simulink model "ATOM_simple_planning_simulator"  (R2026a)
settings: Solver=ode4  StopTime=50  FixedStep=0.01
StopFcn:
  | if exist('costmap_active','var') && ...
  |    exist('vehicle','var') && ...
  |    exist('parking_path','var') && ...
  |    ~isempty(parking_path)
  | 
  |     plotPlan(costmap_active, vehicle, parking_path);
  | else
  |     warning('No valid parking path is available for plotting.');
  | end
model workspace (MAT data in the model file):
  vehicle : object (value not decoded)
symbols that are objects in the model workspace (value not decoded): vehicle
undefined symbols (not defined in the file or in its folder): delta_f_LUT, gain4WS_LUT, k_ref_LUT, kappa_gain_BP, Ki, Kp, lateral, longitudinal, planning_validator, rr_gain_BP, rr_LUT, stanley, velocity_smoother
libraries: slpidlib x1, simulink x1
(part 2 of 7)

== system ATOM_simple_planning_simulator/Parking Scenario/Costmap generation: perpendicular lot ==
  From Workspace1 : FromWorkspace  VariableName=veh
  Perpendicular Parking : MATLAB Function  TreatAsAtomicUnit=on
  costmap : Outport
  start_pose : Outport  Port=2
  goal_pose : Outport  Port=3
  wires:
  Perpendicular Parking/1(costmap) -> costmap/1
  From Workspace1/1 -> Perpendicular Parking/1(veh)
  Perpendicular Parking/2(start_pose) -> start_pose/1
  Perpendicular Parking/3(goal_pose) -> goal_pose/1

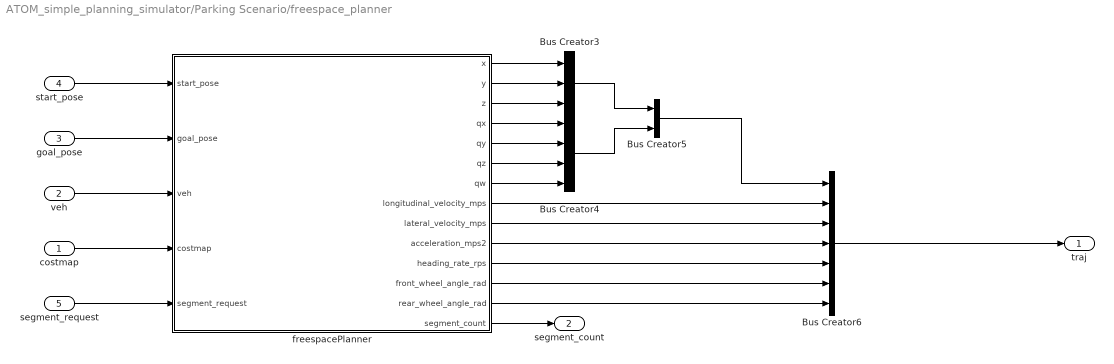
== system ATOM_simple_planning_simulator/Parking Scenario/freespace_planner ==
  costmap : Inport
  veh : Inport  Port=2
  goal_pose : Inport  Port=3
  start_pose : Inport  Port=4
  segment_request : Inport  Port=5
  Bus Creator3 : BusCreator  Inputs=3  OutDataTypeStr=Bus: PointBusN
  Bus Creator4 : BusCreator  Inputs=4  OutDataTypeStr=Bus: QuaternionBusN
  Bus Creator5 : BusCreator  Inputs=2  OutDataTypeStr=Bus: PoseBusN
      settings: InheritFromInputs=off
  Bus Creator6 : BusCreator  Inputs=7  OutDataTypeStr=Bus: TrajectoryDataBus
      settings: InheritFromInputs=off
  freespacePlanner : MATLAB Function  TreatAsAtomicUnit=on
  traj : Outport
  segment_count : Outport  Port=2
  wires:
  Bus Creator6/1 -> traj/1
  Bus Creator3/1 -> Bus Creator5/1
  freespacePlanner/13(rear_wheel_angle_rad) -> Bus Creator6/7
  Bus Creator5/1 -> Bus Creator6/1
  freespacePlanner/8(longitudinal_velocity_mps) -> Bus Creator6/2
  freespacePlanner/3(z) -> Bus Creator3/3
  freespacePlanner/4(qx) -> Bus Creator4/1
  freespacePlanner/9(lateral_velocity_mps) -> Bus Creator6/3
  freespacePlanner/10(acceleration_mps2) -> Bus Creator6/4
  freespacePlanner/5(qy) -> Bus Creator4/2
  freespacePlanner/1(x) -> Bus Creator3/1
  freespacePlanner/2(y) -> Bus Creator3/2
  freespacePlanner/7(qw) -> Bus Creator4/4
  freespacePlanner/6(qz) -> Bus Creator4/3
  freespacePlanner/12(front_wheel_angle_rad) -> Bus Creator6/6
  Bus Creator4/1 -> Bus Creator5/2
  freespacePlanner/11(heading_rate_rps) -> Bus Creator6/5
  costmap/1 -> freespacePlanner/4(costmap)
  start_pose/1 -> freespacePlanner/1(start_pose)
  goal_pose/1 -> freespacePlanner/2(goal_pose)
  veh/1 -> freespacePlanner/3(veh)
  segment_request/1 -> freespacePlanner/5(segment_request)
  freespacePlanner/14(segment_count) -> segment_count/1

== system ATOM_simple_planning_simulator/Plot vehicle/SetStanleyTrajectory ==
  ref_traj : Inport
  ego_pose : Inport  Port=2
  Constant1 : Constant  Value=stanley.traj_resample_dist
  Resample Trajectory : MATLAB Function  TreatAsAtomicUnit=on
  calcLongOffsetToSegment : MATLAB Function  TreatAsAtomicUnit=on
  default : Constant  Value=3
  default1 : Constant  Value=pi/2
  findFirstNearestSegmentIndexWithSoftConstraints : MATLAB Function  TreatAsAtomicUnit=on
  trajectory_out : Outport
  wires:
  ref_traj/1 -> Resample Trajectory/1(trajectory_in), calcLongOffsetToSegment/3(trajectory), findFirstNearestSegmentIndexWithSoftConstraints/1(trajectory)
  Constant1/1 -> Resample Trajectory/2(resample_interval_dist)
  calcLongOffsetToSegment/1(ego_offset_to_segment) -> Resample Trajectory/4(ego_offset_to_segment)
  ego_pose/1 -> findFirstNearestSegmentIndexWithSoftConstraints/4(pose), calcLongOffsetToSegment/2(ego_pose)
  findFirstNearestSegmentIndexWithSoftConstraints/1(nearest_seg_idx) -> calcLongOffsetToSegment/1(seg_idx), Resample Trajectory/3(nearest_seg_idx)
  default/1 -> findFirstNearestSegmentIndexWithSoftConstraints/2(dist_threshold)
  default1/1 -> findFirstNearestSegmentIndexWithSoftConstraints/3(yaw_threshold)
  Resample Trajectory/1(trajectory_out) -> trajectory_out/1

== system ATOM_simple_planning_simulator/Plot vehicle1/SetStanleyTrajectory ==
  ref_traj : Inport
  ego_pose : Inport  Port=2
  Constant1 : Constant  Value=stanley.traj_resample_dist
  Resample Trajectory : MATLAB Function  TreatAsAtomicUnit=on
  calcLongOffsetToSegment : MATLAB Function  TreatAsAtomicUnit=on
  default : Constant  Value=3
  default1 : Constant  Value=pi/2
  findFirstNearestSegmentIndexWithSoftConstraints : MATLAB Function  TreatAsAtomicUnit=on
  trajectory_out : Outport
  wires:
  ref_traj/1 -> Resample Trajectory/1(trajectory_in), calcLongOffsetToSegment/3(trajectory), findFirstNearestSegmentIndexWithSoftConstraints/1(trajectory)
  Constant1/1 -> Resample Trajectory/2(resample_interval_dist)
  calcLongOffsetToSegment/1(ego_offset_to_segment) -> Resample Trajectory/4(ego_offset_to_segment)
  ego_pose/1 -> findFirstNearestSegmentIndexWithSoftConstraints/4(pose), calcLongOffsetToSegment/2(ego_pose)
  findFirstNearestSegmentIndexWithSoftConstraints/1(nearest_seg_idx) -> calcLongOffsetToSegment/1(seg_idx), Resample Trajectory/3(nearest_seg_idx)
  default/1 -> findFirstNearestSegmentIndexWithSoftConstraints/2(dist_threshold)
  default1/1 -> findFirstNearestSegmentIndexWithSoftConstraints/3(yaw_threshold)
  Resample Trajectory/1(trajectory_out) -> trajectory_out/1

== system ATOM_simple_planning_simulator/Vehicle Model/Vehicle Dynamics ==
  command : Inport
  rear_steer_command : Inport  Port=2
  From Workspace : FromWorkspace  VariableName=veh
  MATLAB Function : MATLAB Function  TreatAsAtomicUnit=on
  state integrator : Subsystem
  IntState : Outport
  wires:
  command/1 -> MATLAB Function/2(command)
  MATLAB Function/1(d_state) -> state integrator/1(d_state)  "d_state"
  state integrator/1(state) -> MATLAB Function/1(state), IntState/1
  From Workspace/1 -> MATLAB Function/3(veh)
  rear_steer_command/1 -> MATLAB Function/4(rear_steering_command)

== system ATOM_simple_planning_simulator/Vehicle Model/Vehicle internal state ==
  IntState : Inport
  Bus Selector : BusSelector  OutputSignals=x,y,yaw,vx,steer_front,steer_rear,acc
  Scope{,1..6} (7 alike) : Scope
      Scope settings: ActiveDisplayYMinimum=-1  ActiveDisplayYMaximum=1
      Scope1 settings: ActiveDisplayYMinimum=-1  ActiveDisplayYMaximum=1
      Scope2 settings: ActiveDisplayYMinimum=-1  ActiveDisplayYMaximum=1  DataLoggingVariableName=ScopeData2
      Scope3 settings: ActiveDisplayYMinimum=-1  ActiveDisplayYMaximum=1  DataLoggingVariableName=ScopeData3
      Scope4 settings: ActiveDisplayYMinimum=-1  ActiveDisplayYMaximum=1  DataLoggingVariableName=ScopeData4
      Scope5 settings: ActiveDisplayYMinimum=-1  ActiveDisplayYMaximum=1  DataLoggingVariableName=ScopeData5
      Scope6 settings: ActiveDisplayYMinimum=-1  ActiveDisplayYMaximum=1  DataLoggingVariableName=ScopeData6
  steer_front : Outport
  steer_rear : Outport  Port=2
  wires:
  Bus Selector/2 -> Scope1/1  "<y>"
  Bus Selector/4 -> Scope3/1  "<vx>"
  Bus Selector/1 -> Scope/1  "<x>"
  Bus Selector/3 -> Scope2/1  "<yaw>"
  Bus Selector/7 -> Scope6/1  "<acc>"
  Bus Selector/5 -> steer_front/1, Scope4/1  "<steer_front>"
  Bus Selector/6 -> steer_rear/1, Scope5/1  "<steer_rear>"
  IntState/1 -> Bus Selector/1

== system ATOM_simple_planning_simulator/Vehicle_Model/Vehicle Dynamics ==
  command : Inport
  rear_steer_command : Inport  Port=2
  From Workspace : FromWorkspace  VariableName=veh
  MATLAB Function : MATLAB Function  TreatAsAtomicUnit=on
  state integrator : Subsystem
  IntState : Outport
  wires:
  command/1 -> MATLAB Function/2(command)
  MATLAB Function/1(d_state) -> state integrator/1(d_state)  "d_state"
  state integrator/1(state) -> MATLAB Function/1(state), IntState/1
  From Workspace/1 -> MATLAB Function/3(veh)
  rear_steer_command/1 -> MATLAB Function/4(rear_steering_command)

== system ATOM_simple_planning_simulator/Vehicle_Model/Vehicle internal state ==
  IntState : Inport
  Bus Selector : BusSelector  OutputSignals=x,y,yaw,vx,steer_front,steer_rear,acc
  Scope{,1..6} (7 alike) : Scope
      Scope settings: ActiveDisplayYMinimum=-1  ActiveDisplayYMaximum=1
      Scope1 settings: ActiveDisplayYMinimum=-1  ActiveDisplayYMaximum=1
      Scope2 settings: ActiveDisplayYMinimum=-1  ActiveDisplayYMaximum=1  DataLoggingVariableName=ScopeData2
      Scope3 settings: ActiveDisplayYMinimum=-1  ActiveDisplayYMaximum=1  DataLoggingVariableName=ScopeData3
      Scope4 settings: ActiveDisplayYMinimum=-1  ActiveDisplayYMaximum=1  DataLoggingVariableName=ScopeData4
      Scope5 settings: ActiveDisplayYMinimum=-1  ActiveDisplayYMaximum=1  DataLoggingVariableName=ScopeData5
      Scope6 settings: ActiveDisplayYMinimum=-1  ActiveDisplayYMaximum=1  DataLoggingVariableName=ScopeData6
  steer_front : Outport
  steer_rear : Outport  Port=2
  wires:
  Bus Selector/2 -> Scope1/1  "<y>"
  Bus Selector/4 -> Scope3/1  "<vx>"
  Bus Selector/1 -> Scope/1  "<x>"
  Bus Selector/3 -> Scope2/1  "<yaw>"
  Bus Selector/7 -> Scope6/1  "<acc>"
  Bus Selector/5 -> steer_front/1, Scope4/1  "<steer_front>"
  Bus Selector/6 -> steer_rear/1, Scope5/1  "<steer_rear>"
  IntState/1 -> Bus Selector/1

== system ATOM_simple_planning_simulator/trajectory_checker plugin - planning_validator_node/check_valid_steering ==
  trajectory : Inport
  veh : Inport  Port=2
  CheckValidSteering : MATLAB Function  TreatAsAtomicUnit=on
  Constant : Constant  Value=planning_validator.steering.threshold
  calcMaxSteeringAngles : Subsystem
  is_valid_steering : Outport
  wires:
  calcMaxSteeringAngles/1(max_steering) -> CheckValidSteering/1(max_steering)
  calcMaxSteeringAngles/2(i) -> ?
  Constant/1 -> CheckValidSteering/2(steering_threshold)
  CheckValidSteering/1(is_valid_steering) -> is_valid_steering/1
  trajectory/1 -> calcMaxSteeringAngles/1(trajectory)
  veh/1 -> calcMaxSteeringAngles/2(veh)

== system ATOM_simple_planning_simulator/trajectory_checker plugin - planning_validator_node/check_valid_steering_rate ==
  trajectory : Inport
  veh : Inport  Port=2
  CheckValidSteeringRate : MATLAB Function  TreatAsAtomicUnit=on
  Constant : Constant  Value=planning_validator.steering_rate.threshold
  calcMaxSteeringRates : Subsystem
  is_valid_steering_rate : Outport
  wires:
  calcMaxSteeringRates/1(max_steering_rate) -> CheckValidSteeringRate/1(max_steering_rate)
  calcMaxSteeringRates/2(i) -> ?
  Constant/1 -> CheckValidSteeringRate/2(steering_rate_threshold)
  CheckValidSteeringRate/1(is_valid_steering_rate) -> is_valid_steering_rate/1
  trajectory/1 -> calcMaxSteeringRates/1(trajectory)
  veh/1 -> calcMaxSteeringRates/2(veh)

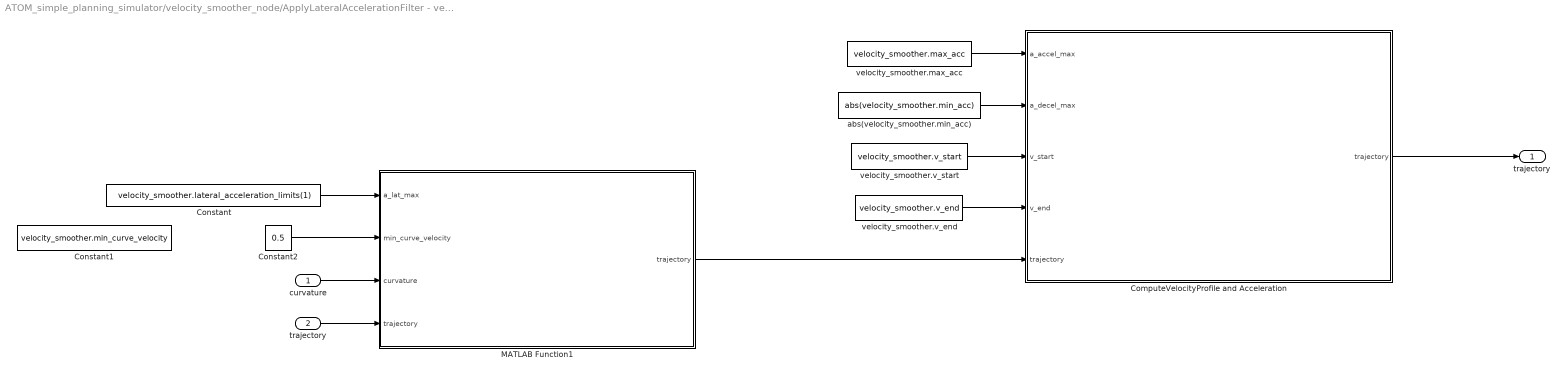
== system ATOM_simple_planning_simulator/velocity_smoother_node/ApplyLateralAccelerationFilter - velocity_smoother node ==
  curvature : Inport
  "trajectory " : Inport  Port=2
  ComputeVelocityProfile and Acceleration : MATLAB Function  TreatAsAtomicUnit=on
  Constant : Constant  Value=velocity_smoother.lateral_acceleration_limits(1)
  Constant1 : Constant  Value=velocity_smoother.min_curve_velocity
  Constant2 : Constant  Value=0.5
  MATLAB Function1 : MATLAB Function  TreatAsAtomicUnit=on
  abs(velocity_smoother.min_acc) : Constant  Value=abs(velocity_smoother.min_acc)
  velocity_smoother.max_acc : Constant  Value=velocity_smoother.max_acc
  velocity_smoother.v_end : Constant  Value=velocity_smoother.v_end
  velocity_smoother.v_start : Constant  Value=velocity_smoother.v_start
  trajectory : Outport
  wires:
  velocity_smoother.v_end/1 -> ComputeVelocityProfile and Acceleration/4(v_end)
  ComputeVelocityProfile and Acceleration/1(trajectory) -> trajectory/1
  curvature/1 -> MATLAB Function1/3(curvature)
  velocity_smoother.v_start/1 -> ComputeVelocityProfile and Acceleration/3(v_start)
  velocity_smoother.max_acc/1 -> ComputeVelocityProfile and Acceleration/1(a_accel_max)
  abs(velocity_smoother.min_acc)/1 -> ComputeVelocityProfile and Acceleration/2(a_decel_max)
  MATLAB Function1/1(trajectory) -> ComputeVelocityProfile and Acceleration/5("trajectory ")
  Constant2/1 -> MATLAB Function1/2(min_curve_velocity)
  Constant/1 -> MATLAB Function1/1(a_lat_max)
  "trajectory "/1 -> MATLAB Function1/4("trajectory ")

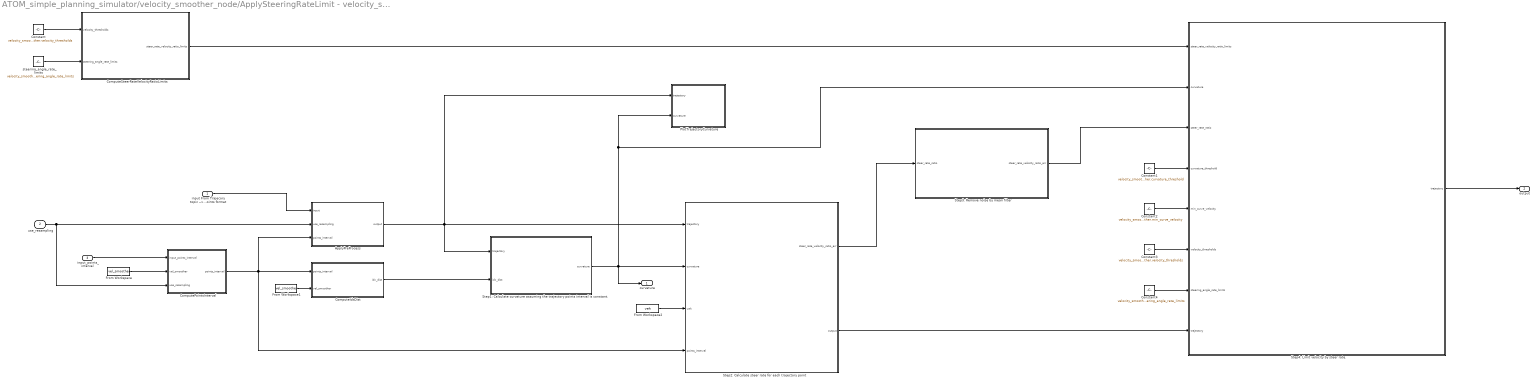
== system ATOM_simple_planning_simulator/velocity_smoother_node/ApplySteeringRateLimit - velocity_smoother_node ==
  input From Trajecory topic --> TrajectoryPoints format : Inport
  use_resampling : Inport  Port=2
  input_points_interval : Inport  Port=3
  ApplyPreProcess : MATLAB Function  TreatAsAtomicUnit=on
  ComputeIdxDist : MATLAB Function  TreatAsAtomicUnit=on
  ComputePointsInterval : MATLAB Function  TreatAsAtomicUnit=on
  ComputeSteerRateVelocityRatioLimits : MATLAB Function  TreatAsAtomicUnit=on
  Constant : Constant  Value=velocity_smoother.velocity_thresholds
  Constant1 : Constant  Value=velocity_smoother.curvature_threshold
  Constant2 : Constant  Value=velocity_smoother.min_curve_velocity
  Constant3 : Constant  Value=velocity_smoother.velocity_thresholds
  Constant4 : Constant  Value=velocity_smoother.steering_angle_rate_limits
  From Workspace : FromWorkspace  VariableName=vel_smoother
  From Workspace1 : FromWorkspace  VariableName=vel_smoother
  From Workspace2 : FromWorkspace  VariableName=veh
  PlotTrajectoryCurvature : MATLAB Function  TreatAsAtomicUnit=on
  Step1: Calculate curvature assuming the trajectory points interval is constant. : Subsystem
  Step2: Calculate steer rate for each trajectory point : Subsystem
  Step3: Remove noise by mean filter : Subsystem
  Step4: Limit velocity by steer rate. : Subsystem
  steering_angle_rate_limits : Constant  Value=velocity_smoother.steering_angle_rate_limits
  curvature : Outport
  output : Outport  Port=2
  wires:
  use_resampling/1 -> ApplyPreProcess/2(use_resempling), ComputePointsInterval/3(use_resampling)
  input From Trajecory topic --> TrajectoryPoints format/1 -> ApplyPreProcess/1(input)
  input_points_interval/1 -> ComputePointsInterval/1(input_points_interval)
  ComputePointsInterval/1(points_interval) -> Step2: Calculate steer rate for each trajectory point/4(points_interval), ComputeIdxDist/1(points_interval), ApplyPreProcess/3(points_interval)
  From Workspace/1 -> ComputePointsInterval/2(vel_smoother)
  From Workspace1/1 -> ComputeIdxDist/2(vel_smoother)
  ApplyPreProcess/1(output) -> PlotTrajectoryCurvature/1(trajectory), Step1: Calculate curvature assuming the trajectory points interval is constant./1(trajectory), Step2: Calculate steer rate for each trajectory point/1(trajectory)
  Step1: Calculate curvature assuming the trajectory points interval is constant./1(curvature) -> curvature/1, PlotTrajectoryCurvature/2(curvature), Step4: Limit velocity by steer rate./2(curvature), Step2: Calculate steer rate for each trajectory point/2(curvature)
  ComputeIdxDist/1(idx_dist) -> Step1: Calculate curvature assuming the trajectory points interval is constant./2(idx_dist)
  From Workspace2/1 -> Step2: Calculate steer rate for each trajectory point/3(veh)
  Step2: Calculate steer rate for each trajectory point/1(steer_rate_velocity_ratio_arr) -> Step3: Remove noise by mean filter/1(steer_rate_ratio)
  steering_angle_rate_limits/1 -> ComputeSteerRateVelocityRatioLimits/2(steering_angle_rate_limits)
  Constant/1 -> ComputeSteerRateVelocityRatioLimits/1(velocity_thresholds)
  ComputeSteerRateVelocityRatioLimits/1(steer_rate_velocity_ratio_limits) -> Step4: Limit velocity by steer rate./1(steer_rate_velocity_ratio_limits)
  Step3: Remove noise by mean filter/1(steer_rate_velocity_ratio_arr) -> Step4: Limit velocity by steer rate./3(steer_rate_ratio)
  Constant1/1 -> Step4: Limit velocity by steer rate./4(curvature_threshold)
  Constant2/1 -> Step4: Limit velocity by steer rate./5(min_curve_velocity)
  Constant3/1 -> Step4: Limit velocity by steer rate./6(velocity_thresholds)
  Constant4/1 -> Step4: Limit velocity by steer rate./7(steering_angle_rate_limits)
  Step2: Calculate steer rate for each trajectory point/2(output) -> Step4: Limit velocity by steer rate./8("trajectory ")
  Step4: Limit velocity by steer rate./1(trajectory) -> output/1

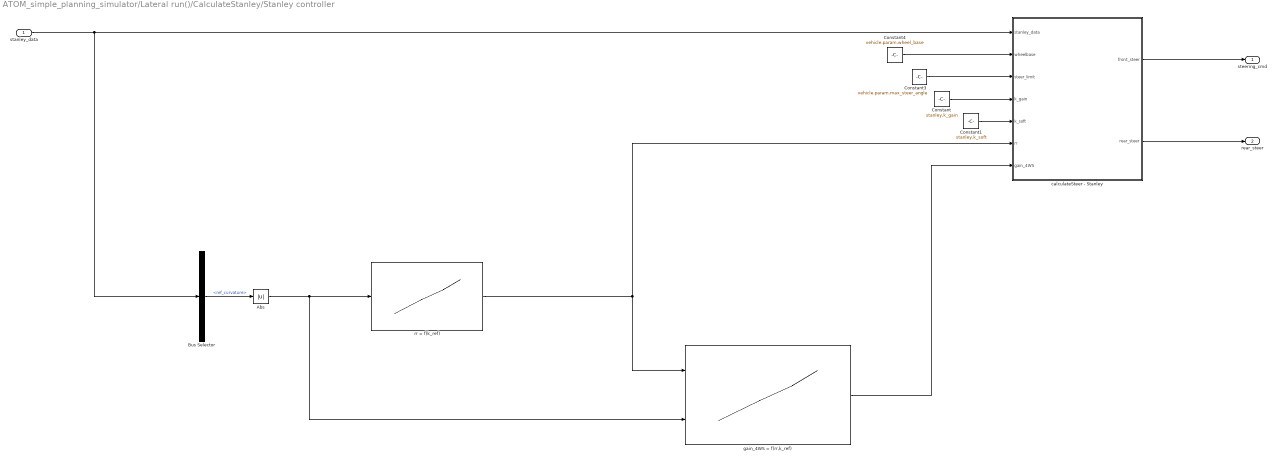
== system ATOM_simple_planning_simulator/Lateral run()/CalculateStanley/Stanley controller ==
  stanley_data : Inport
  Abs : Abs  SaturateOnIntegerOverflow=off
  Bus Selector : BusSelector  OutputSignals=ref_curvature
  Constant : Constant  Value=stanley.k_gain
  Constant1 : Constant  Value=stanley.k_soft
  Constant3 : Constant  Value=vehicle.param.max_steer_angle
  Constant4 : Constant  Value=vehicle.param.wheel_base
  calculateSteer - Stanley : MATLAB Function  TreatAsAtomicUnit=on
  gain_4WS = f(rr,k_ref) : Lookup_n-D  BreakpointsForDimension1=rr_gain_BP  BreakpointsForDimension2=kappa_gain_BP  Table=gain4WS_LUT  InternalRulePriority=Speed  RndMeth=Simplest
      settings: InputPortMap=u0,u1
  rr = f(k_ref) : Lookup_n-D  NumberOfTableDimensions=1  BreakpointsForDimension1=k_ref_LUT  Table=rr_LUT  InternalRulePriority=Speed  RndMeth=Simplest
  steering_cmd : Outport
  rear_steer : Outport  Port=2
  wires:
  Constant1/1 -> calculateSteer - Stanley/5(k_soft)
  Constant/1 -> calculateSteer - Stanley/4(k_gain)
  stanley_data/1 -> calculateSteer - Stanley/1(stanley_data), Bus Selector/1
  calculateSteer - Stanley/1(front_steer) -> steering_cmd/1
  Constant4/1 -> calculateSteer - Stanley/2(wheelbase)
  gain_4WS = f(rr,k_ref)/1 -> calculateSteer - Stanley/7(gain_4WS)
  calculateSteer - Stanley/2(rear_steer) -> rear_steer/1
  Bus Selector/1 -> Abs/1  "<ref_curvature>"
  rr = f(k_ref)/1 -> gain_4WS = f(rr,k_ref)/1, calculateSteer - Stanley/6(rr)
  Constant3/1 -> calculateSteer - Stanley/3(steer_limit)
  Abs/1 -> gain_4WS = f(rr,k_ref)/2, rr = f(k_ref)/1

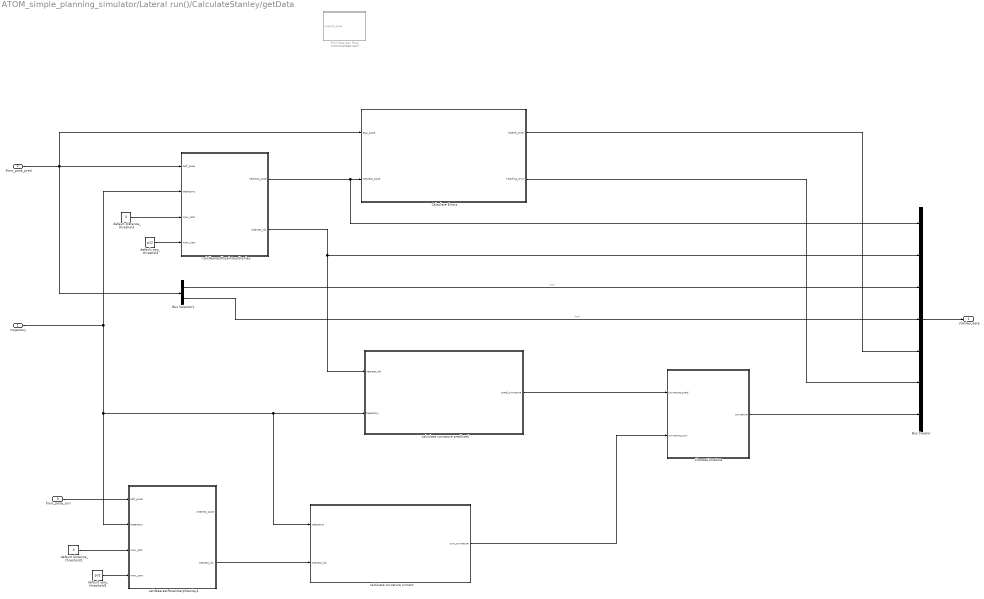
== system ATOM_simple_planning_simulator/Lateral run()/CalculateStanley/getData ==
  trajectory : Inport
  front_pose_pred : Inport  Port=2
  front_pose_curr : Inport  Port=3
  Bus Creator : BusCreator  Inputs=7  OutDataTypeStr=Bus: StanleyInputDataBus
      settings: InheritFromInputs=off
  Bus Selector1 : BusSelector  OutputSignals=twist.linear.x,twist.linear.y
  Calculate Errors : Subsystem
  ChooseCurvature : MATLAB Function  TreatAsAtomicUnit=on
  Plot Nearest Pose : MATLAB Function  Commented=on  TreatAsAtomicUnit=on
  calcNearestPoseInterpStanley : MATLAB Function  TreatAsAtomicUnit=on
  calcNearestPoseInterpStanley1 : MATLAB Function  TreatAsAtomicUnit=on
  calculate curvature current : Subsystem
  calculate curvature predicted : Subsystem
  default distance_threshold : Constant  Value=3
  default distance_threshold1 : Constant  Value=3
  default yaw_threshold : Constant  Value=pi/2
  default yaw_threshold1 : Constant  Value=pi/2
  stanley_data : Outport
  wires:
  default distance_threshold/1 -> calcNearestPoseInterpStanley/3(max_dist)
  default yaw_threshold/1 -> calcNearestPoseInterpStanley/4(max_yaw)
  front_pose_pred/1 -> Bus Selector1/1, Calculate Errors/1(ego_pose), calcNearestPoseInterpStanley/1(self_pose)
  calcNearestPoseInterpStanley/2(nearest_idx) -> calculate curvature predicted/1(nearest_idx), Bus Creator/2
  Bus Creator/1 -> stanley_data/1
  Bus Selector1/1 -> Bus Creator/3  "<x>"
  Calculate Errors/1(lateral_error) -> Bus Creator/5
  Calculate Errors/2(heading_error) -> Bus Creator/6
  calculate curvature predicted/1(pred_curvature) -> ChooseCurvature/1(curvature_pred)
  front_pose_curr/1 -> calcNearestPoseInterpStanley1/1(self_pose)
  default distance_threshold1/1 -> calcNearestPoseInterpStanley1/3(max_dist)
  default yaw_threshold1/1 -> calcNearestPoseInterpStanley1/4(max_yaw)
  calcNearestPoseInterpStanley1/2(nearest_idx) -> calculate curvature current/2(nearest_idx)
  trajectory/1 -> calcNearestPoseInterpStanley/2(trajectory), calcNearestPoseInterpStanley1/2(trajectory), calculate curvature current/1(trajectory), calculate curvature predicted/2(trajectory)
  calculate curvature current/1(curr_curvature) -> ChooseCurvature/2(curvature_curr)
  ChooseCurvature/1(curvature) -> Bus Creator/7
  calcNearestPoseInterpStanley/1(nearest_pose) -> Bus Creator/1, Calculate Errors/2(nearest_pose)
  Bus Selector1/2 -> Bus Creator/4  "<y>"

== system ATOM_simple_planning_simulator/Vehicle Model/Vehicle Dynamics/state integrator ==
  d_state : Inport
  Bus Creator : BusCreator  Inputs=7  OutDataTypeStr=Bus: VehicleInternalStateBus
      settings: InheritFromInputs=off
  Bus Selector : BusSelector  OutputSignals=acc,steer_rear,steer_front,vx,yaw,y,x
  Integrator{,1..5} (6 alike) : Integrator
  Integrator6 : Integrator  InitialCondition=-2
  state : Outport
  wires:
  Integrator4/1 -> Bus Creator/3
  Integrator3/1 -> Bus Creator/4
  Integrator6/1 -> Bus Creator/1
  Bus Selector/4 -> Integrator3/1  "<vx>"
  Integrator1/1 -> Bus Creator/6
  Bus Creator/1 -> state/1
  Bus Selector/6 -> Integrator5/1  "<y>"
  Bus Selector/2 -> Integrator1/1  "<steer_rear>"
  Integrator5/1 -> Bus Creator/2
  Bus Selector/7 -> Integrator6/1  "<x>"
  Bus Selector/3 -> Integrator2/1  "<steer_front>"
  Bus Selector/1 -> Integrator/1  "<acc>"
  Integrator/1 -> Bus Creator/7
  Bus Selector/5 -> Integrator4/1  "<yaw>"
  d_state/1 -> Bus Selector/1
  Integrator2/1 -> Bus Creator/5

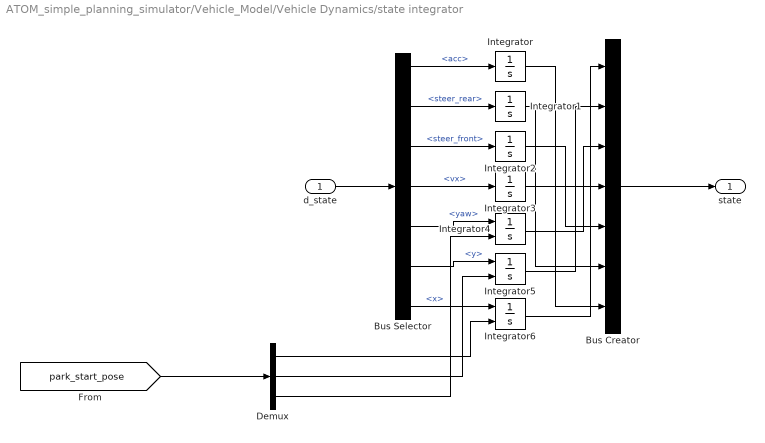
== system ATOM_simple_planning_simulator/Vehicle_Model/Vehicle Dynamics/state integrator ==
  d_state : Inport
  Bus Creator : BusCreator  Inputs=7  OutDataTypeStr=Bus: VehicleInternalStateBus
      settings: InheritFromInputs=off
  Bus Selector : BusSelector  OutputSignals=acc,steer_rear,steer_front,vx,yaw,y,x
  Demux : Demux  Outputs=3
  Integrator{,1..3} (4 alike) : Integrator
  Integrator4 : Integrator  InitialConditionSource=external
  Integrator5 : Integrator  InitialConditionSource=external
  Integrator6 : Integrator  InitialConditionSource=external  InitialCondition=-2
  state : Outport
  wires:
  Integrator4/1 -> Bus Creator/3
  Integrator3/1 -> Bus Creator/4
  Integrator6/1 -> Bus Creator/1
  Bus Selector/4 -> Integrator3/1  "<vx>"
  Integrator1/1 -> Bus Creator/6
  Bus Creator/1 -> state/1
  Bus Selector/6 -> Integrator5/1  "<y>"
  Bus Selector/2 -> Integrator1/1  "<steer_rear>"
  Integrator5/1 -> Bus Creator/2
  Bus Selector/7 -> Integrator6/1  "<x>"
  Bus Selector/3 -> Integrator2/1  "<steer_front>"
  Bus Selector/1 -> Integrator/1  "<acc>"
  Integrator/1 -> Bus Creator/7
  Bus Selector/5 -> Integrator4/1  "<yaw>"
  d_state/1 -> Bus Selector/1
  Integrator2/1 -> Bus Creator/5
  [park_start_pose] -> Demux/1
  Demux/1 -> Integrator6/2
  Demux/2 -> Integrator5/2
  Demux/3 -> Integrator4/2

== system ATOM_simple_planning_simulator/trajectory_checker plugin - planning_validator_node/check_valid_steering/calcMaxSteeringAngles ==
  trajectory : Inport
  veh : Inport  Port=2
  DecideValIdx : MATLAB Function  TreatAsAtomicUnit=on
  GetAbsMaxValAndIdx front : MATLAB Function  TreatAsAtomicUnit=on
  GetAbsMaxValAndIdx rear : MATLAB Function  TreatAsAtomicUnit=on
  calcSteeringAngles : Subsystem
  max_steering : Outport
  i : Outport  Port=2
  wires:
  trajectory/1 -> calcSteeringAngles/1(trajectory)
  veh/1 -> calcSteeringAngles/2(veh)
  calcSteeringAngles/2(rear_steering_vector) -> GetAbsMaxValAndIdx rear/1(values)
  calcSteeringAngles/1(front_steering_vector) -> GetAbsMaxValAndIdx front/1(values)
  GetAbsMaxValAndIdx front/1(max_value) -> DecideValIdx/1(max_front)
  GetAbsMaxValAndIdx rear/2(max_index) -> DecideValIdx/4(idx_rear)
  GetAbsMaxValAndIdx rear/1(max_value) -> DecideValIdx/3(max_rear)
  GetAbsMaxValAndIdx front/2(max_index) -> DecideValIdx/2(idx_front)
  DecideValIdx/1(max_steering) -> max_steering/1
  DecideValIdx/2(max_index) -> i/1

== system ATOM_simple_planning_simulator/trajectory_checker plugin - planning_validator_node/check_valid_steering_rate/calcMaxSteeringRates ==
  trajectory : Inport
  veh : Inport  Port=2
  DecideValIdx : MATLAB Function  TreatAsAtomicUnit=on
  MATLAB Function : MATLAB Function  TreatAsAtomicUnit=on
  MATLAB Function1 : MATLAB Function  TreatAsAtomicUnit=on
  calcSteeringAngles : Subsystem
  max_steering_rate : Outport
  i : Outport  Port=2
  wires:
  trajectory/1 -> MATLAB Function1/1(trajectory), MATLAB Function/1(trajectory), calcSteeringAngles/1(trajectory)
  veh/1 -> calcSteeringAngles/2(veh)
  DecideValIdx/1(max_steering_rate) -> max_steering_rate/1
  DecideValIdx/2(max_index) -> i/1
  calcSteeringAngles/1(front_steering_vector) -> MATLAB Function/2(steering_vector)
  calcSteeringAngles/2(rear_steering_vector) -> MATLAB Function1/2(steering_vector)
  MATLAB Function/1(max_steering_rate) -> DecideValIdx/1(max_front)
  MATLAB Function/2(max_index) -> DecideValIdx/2(idx_front)
  MATLAB Function1/1(max_steering_rate) -> DecideValIdx/3(max_rear)
  MATLAB Function1/2(max_index) -> DecideValIdx/4(idx_rear)

== system ATOM_simple_planning_simulator/velocity_smoother_node/ApplySteeringRateLimit - velocity_smoother_node/Step1: Calculate curvature assuming the trajectory points interval is constant. ==
  trajectory : Inport
  idx_dist : Inport  Port=2
  CalcTrajectoryCurvature : MATLAB Function  TreatAsAtomicUnit=on
  curvature : Outport
  wires:
  idx_dist/1 -> CalcTrajectoryCurvature/2(idx_dist)
  CalcTrajectoryCurvature/1(curvature) -> curvature/1
  trajectory/1 -> CalcTrajectoryCurvature/1(trajectory)

== system ATOM_simple_planning_simulator/velocity_smoother_node/ApplySteeringRateLimit - velocity_smoother_node/Step2: Calculate steer rate for each trajectory point ==
  trajectory : Inport
  curvature : Inport  Port=2
  veh : Inport  Port=3
  points_interval : Inport  Port=4
  ComputeSteeringRate4WS : MATLAB Function  TreatAsAtomicUnit=on
  Constant : Constant  Value=k_ref_LUT
  Constant1 : Constant  Value=rr_LUT
  Constant2 : Constant  Value=delta_f_LUT
  steer_rate_velocity_ratio_arr : Outport
  output : Outport  Port=2
  wires:
  curvature/1 -> ComputeSteeringRate4WS/2(curvature)
  trajectory/1 -> ComputeSteeringRate4WS/1(trajectory)
  points_interval/1 -> ComputeSteeringRate4WS/4(points_interval)
  veh/1 -> ComputeSteeringRate4WS/3(veh)
  ComputeSteeringRate4WS/1(steer_rate_velocity_ratio_arr) -> steer_rate_velocity_ratio_arr/1
  ComputeSteeringRate4WS/2(output) -> output/1
  Constant/1 -> ComputeSteeringRate4WS/5(k_ref_LUT)
  Constant1/1 -> ComputeSteeringRate4WS/6(rr_LUT)
  Constant2/1 -> ComputeSteeringRate4WS/7(delta_f_LUT)

== system ATOM_simple_planning_simulator/velocity_smoother_node/ApplySteeringRateLimit - velocity_smoother_node/Step3: Remove noise by mean filter ==
  steer_rate_ratio : Inport
  MeanFilterSteeringRateRato : MATLAB Function  TreatAsAtomicUnit=on
  steer_rate_velocity_ratio_arr : Outport
  wires:
  steer_rate_ratio/1 -> MeanFilterSteeringRateRato/1(steer_rate_ratio)
  MeanFilterSteeringRateRato/1(steer_rate_velocity_ratio_arr) -> steer_rate_velocity_ratio_arr/1

== system ATOM_simple_planning_simulator/velocity_smoother_node/ApplySteeringRateLimit - velocity_smoother_node/Step4: Limit velocity by steer rate. ==
  steer_rate_velocity_ratio_limits : Inport
  curvature : Inport  Port=2
  steer_rate_ratio : Inport  Port=3
  curvature_threshold : Inport  Port=4
  min_curve_velocity : Inport  Port=5
  velocity_thresholds : Inport  Port=6
  steering_angle_rate_limits : Inport  Port=7
  "trajectory " : Inport  Port=8
  ApplySteeringRateVelocityLimit : MATLAB Function  TreatAsAtomicUnit=on
  trajectory : Outport
  wires:
  velocity_thresholds/1 -> ApplySteeringRateVelocityLimit/6(velocity_thresholds)
  ApplySteeringRateVelocityLimit/1(trajectory) -> trajectory/1
  "trajectory "/1 -> ApplySteeringRateVelocityLimit/8("trajectory ")
  steer_rate_velocity_ratio_limits/1 -> ApplySteeringRateVelocityLimit/1(steer_rate_velocity_ratio_limits)
  curvature/1 -> ApplySteeringRateVelocityLimit/2(curvature)
  steer_rate_ratio/1 -> ApplySteeringRateVelocityLimit/3(steer_rate_ratio)
  steering_angle_rate_limits/1 -> ApplySteeringRateVelocityLimit/7(steering_angle_rate_limits)
  curvature_threshold/1 -> ApplySteeringRateVelocityLimit/4(curvature_threshold)
  min_curve_velocity/1 -> ApplySteeringRateVelocityLimit/5(min_curve_velocity)

== system ATOM_simple_planning_simulator/Lateral run()/CalculateStanley/getData/Calculate Errors ==
  ego_pose : Inport
  nearest_pose : Inport  Port=2
  Plot Stanley Errors : MATLAB Function  TreatAsAtomicUnit=on
  calcLateralErrorStanley : MATLAB Function  TreatAsAtomicUnit=on
  calcYawErrorStanley : MATLAB Function  TreatAsAtomicUnit=on
  lateral_error : Outport
  heading_error : Outport  Port=2
  wires:
  nearest_pose/1 -> calcYawErrorStanley/2(nearest_pose), calcLateralErrorStanley/2(nearest_pose)
  ego_pose/1 -> calcLateralErrorStanley/1(ego_pose), calcYawErrorStanley/1(ego_pose)
  calcYawErrorStanley/1(yaw_err) -> heading_error/1, Plot Stanley Errors/2(heading_error)
  calcLateralErrorStanley/1(lateral_error) -> lateral_error/1, Plot Stanley Errors/1(lateral_error)

== system ATOM_simple_planning_simulator/Lateral run()/CalculateStanley/getData/calculate curvature current ==
  trajectory : Inport
  nearest_idx : Inport  Port=2
  CalcTrajectoryCurvature : MATLAB Function  TreatAsAtomicUnit=on
  ComputeIdxDist : MATLAB Function  TreatAsAtomicUnit=on
  ComputePointsInterval : MATLAB Function  TreatAsAtomicUnit=on
  From Workspace : FromWorkspace  VariableName=vel_smoother
  From Workspace1 : FromWorkspace  VariableName=vel_smoother
  input_points_interval [m] : Constant  OutDataTypeStr=double
  use_resampling == false : Constant  Value=0  OutDataTypeStr=boolean
  curr_curvature : Outport
  wires:
  From Workspace1/1 -> ComputeIdxDist/2(vel_smoother)
  CalcTrajectoryCurvature/1(curvature) -> curr_curvature/1
  use_resampling == false/1 -> ComputePointsInterval/3(use_resampling)
  ComputePointsInterval/1(points_interval) -> ComputeIdxDist/1(points_interval)
  From Workspace/1 -> ComputePointsInterval/2(vel_smoother)
  input_points_interval [m]/1 -> ComputePointsInterval/1(input_points_interval)
  trajectory/1 -> CalcTrajectoryCurvature/1(trajectory)
  ComputeIdxDist/1(idx_dist) -> CalcTrajectoryCurvature/3(idx_dist)
  nearest_idx/1 -> CalcTrajectoryCurvature/2(nearest_idx)

== system ATOM_simple_planning_simulator/Lateral run()/CalculateStanley/getData/calculate curvature predicted ==
  nearest_idx : Inport
  trajectory : Inport  Port=2
  CalcTrajectoryCurvature : MATLAB Function  TreatAsAtomicUnit=on
  ComputeIdxDist : MATLAB Function  TreatAsAtomicUnit=on
  ComputePointsInterval : MATLAB Function  TreatAsAtomicUnit=on
  From Workspace : FromWorkspace  VariableName=vel_smoother
  From Workspace1 : FromWorkspace  VariableName=vel_smoother
  input_points_interval [m] : Constant  OutDataTypeStr=double
  use_resampling == false : Constant  Value=0  OutDataTypeStr=boolean
  pred_curvature : Outport
  wires:
  From Workspace1/1 -> ComputeIdxDist/2(vel_smoother)
  CalcTrajectoryCurvature/1(curvature) -> pred_curvature/1
  use_resampling == false/1 -> ComputePointsInterval/3(use_resampling)
  ComputePointsInterval/1(points_interval) -> ComputeIdxDist/1(points_interval)
  From Workspace/1 -> ComputePointsInterval/2(vel_smoother)
  input_points_interval [m]/1 -> ComputePointsInterval/1(input_points_interval)
  trajectory/1 -> CalcTrajectoryCurvature/1(trajectory)
  ComputeIdxDist/1(idx_dist) -> CalcTrajectoryCurvature/3(idx_dist)
  nearest_idx/1 -> CalcTrajectoryCurvature/2(nearest_idx)

== system ATOM_simple_planning_simulator/trajectory_checker plugin - planning_validator_node/check_valid_steering/calcMaxSteeringAngles/calcSteeringAngles ==
  trajectory : Inport
  veh : Inport  Port=2
  calcCurvature : MATLAB Function  TreatAsAtomicUnit=on
  steering_vector calculation : MATLAB Function  TreatAsAtomicUnit=on
  front_steering_vector : Outport
  rear_steering_vector : Outport  Port=2
  wires:
  steering_vector calculation/2(rear_steering_vector) -> rear_steering_vector/1
  veh/1 -> steering_vector calculation/2(veh)
  trajectory/1 -> calcCurvature/1(trajectory)
  calcCurvature/1(curvature_vector) -> steering_vector calculation/1(curvature)
  steering_vector calculation/1(front_steering_vector) -> front_steering_vector/1

== system ATOM_simple_planning_simulator/trajectory_checker plugin - planning_validator_node/check_valid_steering_rate/calcMaxSteeringRates/calcSteeringAngles ==
  trajectory : Inport
  veh : Inport  Port=2
  calcCurvature : MATLAB Function  TreatAsAtomicUnit=on
  steering_vector calculation : MATLAB Function  TreatAsAtomicUnit=on
  front_steering_vector : Outport
  rear_steering_vector : Outport  Port=2
  wires:
  steering_vector calculation/2(rear_steering_vector) -> rear_steering_vector/1
  veh/1 -> steering_vector calculation/2(veh)
  trajectory/1 -> calcCurvature/1(trajectory)
  calcCurvature/1(curvature_vector) -> steering_vector calculation/1(curvature)
  steering_vector calculation/1(front_steering_vector) -> front_steering_vector/1

== matlab function ATOM_simple_planning_simulator/velocity_smoother_node/ApplySteeringRateLimit - velocity_smoother_node/Step1: Calculate curvature assuming the trajectory points interval is constant./CalcTrajectoryCurvature ==
  data: trajectory input Bus: TrajectoryDataBus; curvature output; idx_dist input
function curvature = ComputeTrajectoryCurvature( ...
    trajectory, ...
    idx_dist)

% ComputeTrajectoryCurvature
%
% Computes the geometric curvature of a trajectory using a three-point
% circle fitting method.
%
% This function reproduces the behavior of:
%
% autoware_motion_utils::calcTrajectoryCurvatureFrom3Points()
%
% used inside:
%
% autoware_velocity_smoother
%
% In the original Autoware implementation, the curvature computation:
%
%   curvature = calc_curvature(p0,p1,p2)
%
% is protected by a C++ try/catch block. If the circle fitting fails
% (for example due to degenerate geometry), Autoware keeps the previous
% curvature value.
%
% MATLAB/Simulink code generation does not support try/catch constructs.
% Therefore this implementation assumes that calc_curvature() is robust
% and handles degenerate cases internally.
%
% Inputs
% -------
% trajectory : struct
%
%   MATLAB representation of Autoware TrajectoryPoints.
%
%   Autoware source:
%
%   autoware_motion_utils/src/trajectory/conversion.cpp
%
%   converts:
%
%       autoware_planning_msgs::msg::Trajectory
%
%   into:
%
%       std::vector<autoware_planning_msgs::msg::TrajectoryPoint>
%
%   via:
%
    % std::vector<autoware_planning_msgs::msg::TrajectoryPoint> convertToTrajectoryPointArray(
    % const autoware_planning_msgs::msg::Trajectory & trajectory)
    % {
    %     std::vector<autoware_planning_msgs::msg::TrajectoryPoint> output(trajectory.points.size());
    %     std::copy(trajectory.points.begin(), trajectory.points.end(), output.begin());
    %     return output;
    % }
%
%
%
%   Each trajectory point contains:
%
%       geometry_msgs/msg/Point pose.position
%
%   with:
%
%       x, y, z
%
%   MATLAB representation:
%
%       trajectory.pose.position.x
%       trajectory.pose.position.y
%       trajectory.pose.position.z
%
%
% idx_dist : scalar
%
%   Number of trajectory samples used as offset for the three-point
%   curvature estimation.
%
%   In Autoware:
%
%       idx_dist =
%       max(floor(curvature_calculation_distance / points_interval),1)
%
%
% Output
% -------
% curvature : Nx1 vector
%
%   Estimated trajectory curvature [1/m].

num_points = length(trajectory.pose.position.x);


%% Not enough trajectory points

% Autoware:
%
% if (trajectory.size() < 3)
% {
%     return vector filled with zeros;
% }

if num_points < 3
    curvature = zeros(num_points,1);
    return;
end


%% Limit idx_dist according to trajectory size

% Autoware:
%
% max_idx_dist =
% floor((trajectory.size()-1)/2)
%
% idx_dist =
% max(1,min(idx_dist,max_idx_dist))

max_idx_dist = floor((num_points-1)/2);

idx_dist = max(1,min(idx_dist,max_idx_dist));


%% Initialize curvature vector

% Autoware:
%
% std::vector<double> k_arr(trajectory.size(),0.0);

curvature = zeros(num_points,1);


%% Three-point curvature estimation

% Autoware:
%
% for (size_t i = 1; i + 1 < trajectory.size(); i++)

% MATLAB indexing:
%
% i = 2 ... N-1

for i = 2:num_points-1


    % Select the three points:
    %
    % p0 : idx_dist samples before
    % p1 : current trajectory point
    % p2 : idx_dist samples after
    %
    % Equivalent to Autoware:
    %
    % p0 = get_point(
    %       trajectory.at(i - min(idx_dist,i)))
    %
    % p1 = get_point(
    %       trajectory.at(i))
    %
    % p2 = get_point(
    %       trajectory.at(
    %       i + min(idx_dist,size-i-1)))


    idx_prev = i - min(idx_dist,i-1);

    idx_curr = i;

    idx_next = i + min(idx_dist,num_points-i);


    % geometry_msgs/msg/Point:
    %
    % float64 x
    % float64 y
    % float64 z

    p0 = [
        trajectory.pose.position.x(idx_prev), ...
        trajectory.pose.position.y(idx_prev), ...
        trajectory.pose.position.z(idx_prev)
        ];

    p1 = [
        trajectory.pose.position.x(idx_curr), ...
        trajectory.pose.position.y(idx_curr), ...
        trajectory.pose.position.z(idx_curr)
        ];

    p2 = [
        trajectory.pose.position.x(idx_next), ...
        trajectory.pose.position.y(idx_next), ...
        trajectory.pose.position.z(idx_next)
        ];


    %% Compute curvature

    % Autoware:
    %
    % try
    % {
    %     curvature = calc_curvature(p0,p1,p2);
    % }
    %
    % catch(...)
    % {
    %     curvature = previous curvature;
    % }
    %
    % try/catch removed because unsupported by Simulink Coder.

    curvature(i) = calc_curvature(p0,p1,p2);


end


%% Boundary curvature completion

% Autoware:
%
% k_arr.at(0) = k_arr.at(1);
% k_arr.back() = k_arr.at(size-2);

curvature(1) = curvature(2);

curvature(end) = curvature(end-1);


end

== matlab function ATOM_simple_planning_simulator/velocity_smoother_node/ApplySteeringRateLimit - velocity_smoother_node/Step4: Limit velocity by steer rate./ApplySteeringRateVelocityLimit ==
  data: steer_rate_velocity_ratio_limits input; curvature input; steer_rate_ratio input; curvature_threshold input; min_curve_velocity input; velocity_thresholds input; steering_angle_rate_limits input; trajectory input Bus: TrajectoryDataBus; trajectory output
function trajectory = ApplySteeringRateVelocityLimit( ...
    steer_rate_velocity_ratio_limits, ...
    curvature, ...
    steer_rate_ratio, ...
    curvature_threshold, ...
    min_curve_velocity, ...
    velocity_thresholds, ...
    steering_angle_rate_limits, ...
    trajectory)

% ApplySteeringRateVelocityLimit
%
% Applies the steering-rate velocity constraint to the trajectory.
%
% Equivalent to Step 4 of:
%
%   SmootherBase::applySteeringRateLimit()
%
% in Autoware.
%
%
% The steering rate itself does not directly modify the steering angles.
% Instead, it generates a local maximum admissible velocity.
%
% Whenever the current trajectory speed exceeds this limit,
% the trajectory longitudinal velocity is reduced.
%
%
% This algorithm is identical for both 2WS and 4WS.
%
% The only difference is how steer_rate_ratio has been computed.
%
%
% In C++, the following reference:
%
%   auto & velocity =
%       output.at(i+k).longitudinal_velocity_mps;
%
% directly modifies the trajectory.
%
% MATLAB has no equivalent reference semantics, therefore the trajectory
% structure is explicitly updated.



N = length(trajectory.longitudinal_velocity_mps);


for i = 1:N-1

    %% Ignore almost straight segments

    if abs(curvature(i)) < curvature_threshold
        continue
    end


    %% Mean velocity

    mean_velocity = ...
        ( ...
        trajectory.longitudinal_velocity_mps(i) + ...
        trajectory.longitudinal_velocity_mps(i+1) ...
        ) / 2;


    %% Local steering-rate velocity limit

    local_velocity_limit = ...
        ComputeVelocityLimitFromSteerRate( ...
        steer_rate_ratio(i), ...
        steer_rate_velocity_ratio_limits, ...
        velocity_thresholds, ...
        steering_angle_rate_limits);

    %% If the following condition is true, do nothing and pass to the next iteration

    if mean_velocity < local_velocity_limit
        continue
    end


    %% Update the two neighbouring trajectory points

    % Equivalent in C++ to:
    % for (size_t k = 0; k < 2; k++) {
    %     auto & velocity = output.at(i+k).longitudinal_velocity_mps;
    % 
    %     const float target_velocity =
    %     std::max(
    %     min_curve_velocity,
    %     std::min(
    %     local_velocity_limit,
    %     velocity * (local_velocity_limit / mean_vel)));
    % 
    %     velocity = std::min(velocity,target_velocity);
    %     }

    for k = 0:1

        idx = i + k;

        velocity = ...
            trajectory.longitudinal_velocity_mps(idx);


        target_velocity = max( ...
            min_curve_velocity, ...
            min( ...
                local_velocity_limit, ...
                velocity * ...
                (local_velocity_limit / mean_velocity)));


        trajectory.longitudinal_velocity_mps(idx) = ...
            min(velocity, target_velocity);

    end

end

end

== matlab function ATOM_simple_planning_simulator/velocity_smoother_node/ApplySteeringRateLimit - velocity_smoother_node/Step2: Calculate steer rate for each trajectory point/ComputeSteeringRate4WS ==
  data: trajectory input Bus: TrajectoryDataBus; curvature input; veh input; steer_rate_velocity_ratio_arr output; points_interval input; output output Bus: TrajectoryDataBus; k_ref_LUT input; rr_LUT input; delta_f_LUT input
function [steer_rate_velocity_ratio_arr, output] = ComputeSteeringRateAngle4WS(trajectory, ...
    curvature, veh, ...
    points_interval, ...
    k_ref_LUT, rr_LUT, delta_f_LUT)


% ComputeSteeringRateAngle4WS
%
% Computes steering angle rate ratio for 4WS.
%
% Equivalent to Autoware:
%
% steer_rate_velocity_ratio_arr
%
%
% The returned value represents:
%
%       steering_angle_difference / distance
%
%
% For 4WS:
%
% front and rear steering rates are computed.
%
% The maximum steering variation is used as constraint.


N = length(curvature);

rr = zeros(N,1);
front_angle = zeros(N,1);
rear_angle  = zeros(N,1);


%% Compute steering angles

for i = 1:N
    
    if curvature(i) > max(k_ref_LUT)
        rr(i) = -1;
        front_angle(i) = 0.7;
        rear_angle(i) = -0.7;
    else                                                         % Modified for 4WS
        rr(i) = interp1(k_ref_LUT, rr_LUT, curvature(i));
        front_angle(i) = interp1(k_ref_LUT, delta_f_LUT, curvature(i));
        rear_angle(i) = rr(i) * front_angle(i);      
    end
end

% This is a collateral effect of (&) in C++ when (considering in original
% Autoware):
%
% auto & steer_front = output.at(i + 1).front_wheel_angle_rad;
% auto & steer_back = output.at(i).front_wheel_angle_rad;
% 
% // calculate the just 2 steering angle
% steer_front = std::atan(base_param_.wheel_base * curvature_v.at(i + 1));
% steer_back = std::atan(base_param_.wheel_base * curvature_v.at(i));
% Indeed, updating steer_front we popolate also output.at(i + 1).front_wheel_angle_rad, 
% and so the output topic is populated (but it's just a collateral effect, front_wheel_angle_rad 
% and rear_wheel_angle_rad contents are not important for Control module.

trajectory.front_wheel_angle_rad = front_angle;
trajectory.rear_wheel_angle_rad  = rear_angle;

%% Compute steering rate

steer_rate_velocity_ratio_arr = zeros(N,1);


for i = 1:N-1


    % auto & steer_front = output.at(i + 1).front_wheel_angle_rad;
    % auto & steer_back = output.at(i).front_wheel_angle_rad;
    % const auto steering_diff = std::fabs(steer_front - steer_back);
    front_diff = abs( ...
        front_angle(i+1)-front_angle(i));


    rear_diff = abs( ...
        rear_angle(i+1)-rear_angle(i));


    steering_diff = max( ...                                    % Modified for 4WS --> conservative solution
        front_diff,...
        rear_diff);

    % eps avoids division by zero:
    eps = 2.220446049250313e-16;

    steer_rate_velocity_ratio_arr(i)= ...
        steering_diff/(points_interval+eps);


end


steer_rate_velocity_ratio_arr(end)= ...
    steer_rate_velocity_ratio_arr(end-1);


% Output topic now presents front_wheel_angle_rad and rear_wheel_angle_rad
% populated
output = trajectory;


end

== matlab function ATOM_simple_planning_simulator/velocity_smoother_node/ApplySteeringRateLimit - velocity_smoother_node/Step3: Remove noise by mean filter/MeanFilterSteeringRateRato ==
  data: steer_rate_ratio input; steer_rate_velocity_ratio_arr output
function steer_rate_velocity_ratio_arr = MeanFilterSteeringRateRatio( ...
    steer_rate_ratio)

% MeanFilterSteeringRateRatio
%
% Applies the same moving-average filter used by Autoware on the steering
% rate ratio.
%
% Equivalent to Step 3 inside:
%
%   SmootherBase::applySteeringRateLimit()
%
% in:
%
%   autoware_velocity_smoother
%
%
% Original C++ implementation:
%
% for (size_t i = 1; i < steer_rate_velocity_ratio_arr.size() - 1; i++) {
%
%   steer_rate_velocity_ratio_arr.at(i) =
%     (steer_rate_velocity_ratio_arr.at(i-1) +
%      steer_rate_velocity_ratio_arr.at(i)   +
%      steer_rate_velocity_ratio_arr.at(i+1))
%      / 3.0;
%
% }
%
%
% Notes
% -----
%
% The filter is performed in-place, exactly as in Autoware.
%
% Consequently, when computing sample i, the previous sample
% (i-1) has already been filtered, while the next sample (i+1)
% is still the original one.
%
% This behaviour is intentionally preserved to remain identical
% to the C++ implementation.


N = length(steer_rate_ratio);

steer_rate_velocity_ratio_arr = zeros(N,1);

for i = 2:N-1

    steer_rate_velocity_ratio_arr(i) = ...
        ( ...
        steer_rate_ratio(i-1) + ...
        steer_rate_ratio(i)   + ...
        steer_rate_ratio(i+1) ...
        ) / 3.0;

end


end

== matlab function ATOM_simple_planning_simulator/velocity_smoother_node/ApplySteeringRateLimit - velocity_smoother_node/ComputePointsInterval ==
  data: input_points_interval input; vel_smoother input; use_resampling input; points_interval output
function points_interval = computePointsInterval(input_points_interval, ...
    vel_smoother, use_resampling)

% Compute the trajectory points interval used for preprocessing.
%
% If resampling is enabled, a constant spatial interval is imposed.
% Otherwise, the original trajectory point spacing is preserved.

sample_ds = vel_smoother(3,1);

if use_resampling

    points_interval = sample_ds;

else

    points_interval = input_points_interval;

end

end

== matlab function ATOM_simple_planning_simulator/velocity_smoother_node/ApplySteeringRateLimit - velocity_smoother_node/ComputeIdxDist ==
  data: points_interval input; idx_dist output; vel_smoother input
function idx_dist = ComputeIdxDist( ...
    points_interval, ...
    vel_smoother)

% ComputeIdxDist
%
% Computes the point offset used for trajectory curvature estimation.
%
% The curvature is evaluated using three trajectory points separated by a
% fixed physical distance. Since the trajectory is sampled with a constant
% spatial interval (points_interval), this function converts the desired
% curvature calculation distance into the corresponding point index offset.
%
% In other words, idx_dist represents the number of trajectory points
% corresponding to the specified curvature calculation distance.
%
% Equivalent to the Autoware implementation:
%
% idx_dist = max(int(curvature_calculation_distance / points_interval), 1);

curvature_calculation_distance = vel_smoother(1);

idx_dist = max( ...
    floor(curvature_calculation_distance / points_interval), ...
    1);

== matlab function ATOM_simple_planning_simulator/velocity_smoother_node/ApplySteeringRateLimit - velocity_smoother_node/PlotTrajectoryCurvature ==
  data: trajectory input; curvature input
function PlotTrajectoryCurvature(trajectory, curvature)

% PlotTrajectoryCurvature
%
% Visualizes the trajectory curvature computed by:
%
%   ComputeTrajectoryCurvature()
%
% Equivalent to inspecting:
%
%   std::vector<double> k_arr
%
% generated inside:
%
%   autoware_motion_utils::calcTrajectoryCurvatureFrom3Points()
%
%
% Inputs
% -------
%
% trajectory:
%   MATLAB representation of Autoware TrajectoryPoints:
%
%       trajectory.pose.position.x
%       trajectory.pose.position.y
%
%
% curvature:
%   Nx1 signed curvature vector [1/m].
%
%   Positive curvature  -> left turn
%   Negative curvature  -> right turn


persistent hCurvature
persistent hTraj


%% Extract trajectory position

x = trajectory.pose.position.x;
y = trajectory.pose.position.y;


%% Check dimensions

if length(curvature) ~= length(x)

    error("Curvature vector length does not match trajectory length.");

end


%% Curvature profile

if isempty(hCurvature) 

    figure(3)
    clf

    hold on
    grid on

    hCurvature = plot( ...
        curvature, ...
        'LineWidth',1.5);


    xlabel("Trajectory point index");
    ylabel("Curvature [1/m]");

    title("Curvature profile");


else

    set(hCurvature,...
        'YData',curvature);

end



%% XY trajectory colored by curvature

if isempty(hTraj) 

    figure(4)
    clf

    hold on
    grid on
    axis equal


    hTraj = scatter( ...
        x, ...
        y, ...
        25, ...
        curvature, ...
        'filled');


    xlabel("x [m]");
    ylabel("y [m]");

    title("Trajectory curvature map");


    cb = colorbar;
    ylabel(cb,'Curvature [1/m]');


else

    set(hTraj,...
        'XData',x,...
        'YData',y,...
        'CData',curvature);

end


drawnow limitrate


end
